simulink model "mass_spring_damper_DMDc"  (R2019b)
settings: Solver=FixedStepAuto  StartTime=0.0  StopTime=200  FixedStep=0.001  RelTol=1e-3
settings Model: PacingRate=3  Creator=Murray  LastModifiedBy=Murray
settings SolverCC: AlgebraicLoopSolver=LineSearch

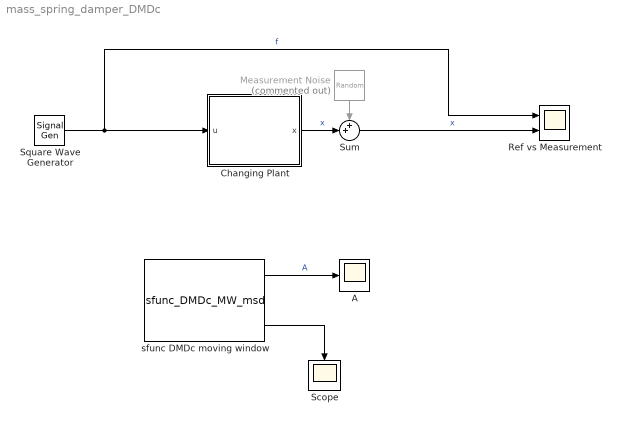
== system mass_spring_damper_DMDc ==
  A : Scope
  Changing Plant : Subsystem
  Measurement Noise : RandomNumber  Commented=on  Variance=0.001  SampleTime=0.05
  Ref vs Measurement : Scope  NumInputPorts=2
  Scope : Scope
  Square Wave Generator : SignalGenerator  WaveForm=square  Frequency=1/20
  Sum : Sum  Inputs=++|
  sfunc DMDc moving window : M-S-Function  FunctionName=sfunc_DMDc_MW_msd  Parameters=30/0.05, 0.05, 30/0.05
      mask Display:
      | port_label('input', 1, 'f')
      | port_label('input', 2, 'x')
      | port_label('input', 3, 'x_dot')
      | port_label('output', 1, 'A')
      | port_label('output', 2, 'B')
      | port_label('output', 3, 'MSE')
  wires:
  Square Wave Generator/1 -> Ref vs Measurement/1, Changing Plant/1(u)  "f"
  Measurement Noise/1 -> Sum/1
  Changing Plant/1(x) -> Sum/2  "x"
  sfunc DMDc moving window/1 -> A/1  "A"
  sfunc DMDc moving window/3 -> Scope/1
  Sum/1 -> Ref vs Measurement/2  "x"

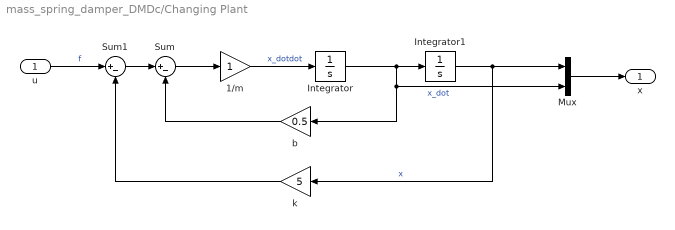
== system mass_spring_damper_DMDc/Changing Plant ==
  u : Inport
  1/m : Gain
  Integrator : Integrator
  Integrator1 : Integrator
  Mux : Mux  Inputs=2
  Sum : Sum  Inputs=|+-
  Sum1 : Sum  Inputs=|+-
  b : Gain  Gain=0.5
  k : Gain  Gain=5
  x : Outport
  wires:
  u/1 -> Sum1/1  "f"
  Integrator/1 -> b/1, Mux/2, Integrator1/1  "x_dot"
  Sum1/1 -> Sum/1
  1/m/1 -> Integrator/1  "x_dotdot"
  Integrator1/1 -> k/1, Mux/1  "x"
  Sum/1 -> 1/m/1
  b/1 -> Sum/2
  k/1 -> Sum1/2
  Mux/1 -> x/1
